simulink model "MBD_FOC_SENSORLESS_MODEL"  (R2022b)
settings: Solver=FixedStepDiscrete  StartTime=0.0  StopTime=9  FixedStep=.00005  RelTol=1e-3  EnableMultiTasking=on
PostLoadFcn:
  | MBD_FOC_SENSORLESS_DATA;
InitFcn:
  | MBD_FOC_SENSORLESS_DATA;
model workspace (MAT data in the model file):
  mwTaskManagerKernelLatency = 1e-06
values from neighbouring files (symbols this model uses):
  Iq_Ref_openLoop = 0.5    [MBD_FOC_SENSORLESS_DATA.m]
  PI_params = mcb.internal.SetControllerParameters(pmsm,inverter,PU_System,T_pwm,Ts,Ts_speed)    [MBD_FOC_SENSORLESS_DATA.m]
  PU_System = mcb_SetPUSystem(pmsm,inverter)    [MBD_FOC_SENSORLESS_DATA.m]
  PWM1max = 1600    [MBD_FOC_SENSORLESS_DATA.m]
  PWM_frequency = 20e3    (= 20000)    [MBD_FOC_SENSORLESS_DATA.m]
  Speed_Ref_openLoop = 500    [MBD_FOC_SENSORLESS_DATA.m]
  Ts = T_pwm    (= 5e-05)    [MBD_FOC_SENSORLESS_DATA.m]
  Ts_speed = 30*Ts    (= 0.0015)    [MBD_FOC_SENSORLESS_DATA.m]
undefined symbols (not defined in the file or in its folder): DiscIntNeverNeededParam, inverter, pmsm
libraries: mcbcontrolslib x9, simulink x4, slpidlib x3, mcbplantlib x1, autolibpmsmexterior x1
(part 2 of 2)

== system MBD_FOC_SENSORLESS_MODEL/Speed Control/Enable Switch/Codegen/Triggered Subsystem ==
  Trigger : TriggerPort  TriggerType=falling  VariantControl=Variant
  Data Store Write : DataStoreWrite  DataStoreName=Enable  IndexOptions=Index vector (dialog)  Indices=1  OutputSizes=1
  Delay : Delay  DelayLength=1  InitialCondition=0
  NOT : Logic  Operator=NOT  IconShape=distinctive  AllPortsSameDT=off  OutDataTypeStr=boolean
  wires:
  NOT/1 -> Data Store Write/1, Delay/1
  Delay/1 -> NOT/1

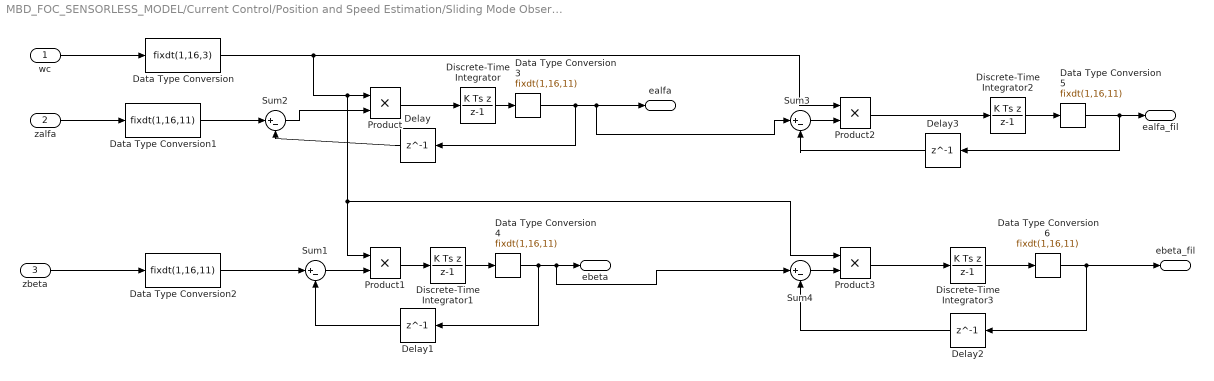
== system MBD_FOC_SENSORLESS_MODEL/Current Control/Position and Speed Estimation/Sliding Mode Observer/SMO Implemetation/Adaptive Filter1 ==
  wc : Inport
  zalfa : Inport  Port=2
  zbeta : Inport  Port=3
  Data Type Conversion : DataTypeConversion  OutDataTypeStr=fixdt(1,16,3)  SaturateOnIntegerOverflow=off  RndMeth=Floor
  Data Type Conversion{1..6} (6 alike) : DataTypeConversion  OutDataTypeStr=fixdt(1,16,11)  SaturateOnIntegerOverflow=off  RndMeth=Floor
  Delay{,1..3} (4 alike) : Delay  DelayLength=1
  Discrete-Time Integrator{,1..3} (4 alike) : DiscreteIntegrator  IntegratorMethod=Integration: Backward Euler  SampleTime=-1  OutDataTypeStr=fixdt(1,32,17)  ICPrevOutput=DiscIntNeverNeededParam  ICPrevScaledInput=DiscIntNeverNeededParam
  Product : Product  OutDataTypeStr=fixdt(1,32,14)
  Product1 : Product  OutDataTypeStr=fixdt(1,32,11)
  Product2 : Product
  Product3 : Product
  Sum{1..4} (4 alike) : Sum  Inputs=|+-
  ealfa : Outport  VectorParamsAs1DForOutWhenUnconnected=off
  ebeta : Outport  Port=2  VectorParamsAs1DForOutWhenUnconnected=off
  ealfa_fil : Outport  Port=3  VectorParamsAs1DForOutWhenUnconnected=off
  ebeta_fil : Outport  Port=4  VectorParamsAs1DForOutWhenUnconnected=off
  wires:
  Sum2/1 -> Product/2
  Product/1 -> Discrete-Time Integrator/1
  zalfa/1 -> Data Type Conversion1/1
  wc/1 -> Data Type Conversion/1
  Product1/1 -> Discrete-Time Integrator1/1
  Sum1/1 -> Product1/2
  zbeta/1 -> Data Type Conversion2/1
  Discrete-Time Integrator1/1 -> Data Type Conversion4/1
  Product2/1 -> Discrete-Time Integrator2/1
  Sum3/1 -> Product2/2
  Discrete-Time Integrator2/1 -> Data Type Conversion5/1
  Discrete-Time Integrator3/1 -> Data Type Conversion6/1
  Sum4/1 -> Product3/2
  Product3/1 -> Discrete-Time Integrator3/1
  Data Type Conversion/1 -> Product3/1, Product1/1, Product/1, Product2/1
  Data Type Conversion1/1 -> Sum2/1
  Data Type Conversion2/1 -> Sum1/1
  Discrete-Time Integrator/1 -> Data Type Conversion3/1
  Data Type Conversion3/1 -> Delay/1, Sum3/1, ealfa/1
  Data Type Conversion4/1 -> Delay1/1, Sum4/1, ebeta/1
  Delay/1 -> Sum2/2
  Delay1/1 -> Sum1/2
  Delay2/1 -> Sum4/2
  Delay3/1 -> Sum3/2
  Data Type Conversion5/1 -> ealfa_fil/1, Delay3/1
  Data Type Conversion6/1 -> ebeta_fil/1, Delay2/1

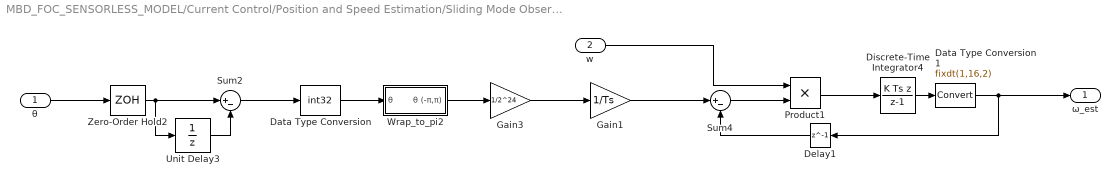
== system MBD_FOC_SENSORLESS_MODEL/Current Control/Position and Speed Estimation/Sliding Mode Observer/SMO Implemetation/Subsystem ==
  θ : Inport
  w : Inport  Port=2
  Data Type Conversion : DataTypeConversion  OutDataTypeStr=int32  ConvertRealWorld=Stored Integer (SI)  SaturateOnIntegerOverflow=off  RndMeth=Floor
  Data Type Conversion1 : DataTypeConversion  OutDataTypeStr=fixdt(1,16,2)  SaturateOnIntegerOverflow=off  RndMeth=Floor
  Delay1 : Delay  DelayLength=1
  Discrete-Time Integrator4 : DiscreteIntegrator  IntegratorMethod=Integration: Backward Euler  SampleTime=-1  OutDataTypeStr=fixdt(1,32,8)  ICPrevOutput=DiscIntNeverNeededParam  ICPrevScaledInput=DiscIntNeverNeededParam
  Gain1 : Gain  Gain=1/Ts  OutDataTypeStr=fixdt(1,16,3)
  Gain3 : Gain  Gain=1/2^24  OutDataTypeStr=fixdt(1,16,12)
  Product1 : Product  OutDataTypeStr=fixdt(1,32,8)
  Sum2 : Sum  Inputs=|+-  AccumDataTypeStr=fixdt(1,16,12)  OutDataTypeStr=fixdt(1,32,24)
  Sum4 : Sum  Inputs=|+-
  Unit Delay3 : UnitDelay  SampleTime=Ts  HasFrameUpgradeWarning=on
  Wrap_to_pi2 : Subsystem  VariantControl=VSS_STD
  Zero-Order Hold2 : ZeroOrderHold  SampleTime=Ts
  ω_est : Outport  VectorParamsAs1DForOutWhenUnconnected=off
  wires:
  Unit Delay3/1 -> Sum2/2
  Zero-Order Hold2/1 -> Sum2/1, Unit Delay3/1
  Wrap_to_pi2/1(θ (-π,π)) -> Gain3/1
  Sum4/1 -> Product1/2
  Product1/1 -> Discrete-Time Integrator4/1
  θ/1 -> Zero-Order Hold2/1
  Gain1/1 -> Sum4/1
  Delay1/1 -> Sum4/2
  Sum2/1 -> Data Type Conversion/1
  Data Type Conversion/1 -> Wrap_to_pi2/1(θ)
  Gain3/1 -> Gain1/1
  Discrete-Time Integrator4/1 -> Data Type Conversion1/1
  w/1 -> Product1/1
  Data Type Conversion1/1 -> Delay1/1, ω_est/1

== system MBD_FOC_SENSORLESS_MODEL/Current Control/Position and Speed Estimation/Sliding Mode Observer/SMO Implemetation/atan2 ==
  note: Consistent with Microchip notation:
      |
      | x_α = cos(θ) * x_d - sin(θ) * x_q
      | x_β = sin(θ) * x_d + cos(θ) * x_q
      |
      | θ = atan2(sin(θ)/cos(θ)) = atan2(-x_α/x_β)
      |
      | provided x_d = 0, which is true in case of E_d
  α : Inport
  β : Inport  Port=2
  Bias2 : Bias  Bias=(pi/4)+(pi/4)  SaturateOnIntegerOverflow=off
  Data Type Conversion3 : DataTypeConversion  OutDataTypeStr=fixdt(1,16,12)  SaturateOnIntegerOverflow=off  RndMeth=Floor
  Data Type Conversion4 : DataTypeConversion  OutDataTypeStr=uint16  ConvertRealWorld=Stored Integer (SI)  SaturateOnIntegerOverflow=off  RndMeth=Floor
  Gain2 : Gain  Gain=1/2^12  OutDataTypeStr=fixdt(1,16,12)
  Gain3 : Gain  Gain=-1  OutDataTypeStr=Inherit: Same as input
  Subsystem1 : Subsystem
  Trigonometric Function : Trigonometry  Operator=atan2  ApproximationMethod=CORDIC
  Wrap_to_pi1 : Subsystem  VariantControl=VSS_STD
  θ : Outport  VectorParamsAs1DForOutWhenUnconnected=off
  wires:
  Trigonometric Function/1 -> Data Type Conversion3/1
  Gain3/1 -> Trigonometric Function/1
  α/1 -> Gain3/1
  β/1 -> Trigonometric Function/2
  Data Type Conversion3/1 -> Subsystem1/1(theta(-pi,pi))
  Subsystem1/1(theta(0,2pi)) -> Bias2/1
  Bias2/1 -> Data Type Conversion4/1
  Data Type Conversion4/1 -> Wrap_to_pi1/1(θ)
  Wrap_to_pi1/1(θ (0,2π)) -> Gain2/1  "z"
  Gain2/1 -> θ/1

== system MBD_FOC_SENSORLESS_MODEL/Current Control/Position and Speed Estimation/Sliding Mode Observer/SMO Implemetation/Subsystem/Wrap_to_pi2 ==
  note: What's left after
      | division by 2pi
  note: This block limits the output angle between +/- π.
  note: Add pi
  note: What's left after
      | division by 2pi
      | again
  note: Subtract pi
  θ : Inport
  Bias : Bias  Bias=pi*16777216  SaturateOnIntegerOverflow=off
  Bias1 : Bias  Bias=-pi*16777216  SaturateOnIntegerOverflow=off
  Math Function : Math  Operator=mod  SignedPower=on
  Math Function1 : Math  Operator=mod  SignedPower=on
  load torque1 : Constant  Value=2*pi*16777216  OutDataTypeStr=int32  SampleTime=Ts
  θ (-π,π) : Outport  VectorParamsAs1DForOutWhenUnconnected=off
  wires:
  Math Function1/1 -> Bias/1
  θ/1 -> Math Function1/1
  Math Function/1 -> Bias1/1
  load torque1/1 -> Math Function1/2, Math Function/2
  Bias/1 -> Math Function/1
  Bias1/1 -> θ (-π,π)/1

== system MBD_FOC_SENSORLESS_MODEL/Current Control/Position and Speed Estimation/Sliding Mode Observer/SMO Implemetation/atan2/Subsystem1 ==
  theta(-pi,pi) : Inport
  2pi : Constant  Value=2*pi  OutDataTypeStr=fixdt(1,16,12)  SampleTime=Ts  mask(TL_Constant){data={'date',734873.5078369329}}
      settings: CopyFcn=if exist('tl_reset_reviewflag','file')==2,tl_reset_reviewflag(gcbh);end  DeleteFcn=if exist('delete_tlblock','file')==2,delete_tlblock(gcbh);end  NameChangeFcn=if exist('rename_tlblock','file')==2,rename_tlblock(gcbh);end  OpenFcn=if exist('tl_open_blockdlg','file')==2,tl_open_blockdlg(gcbh);else,open_system(gcbh,'parameter');end
      mask Help: eval(['if exist(''tl_online_help'',''file'') == 2, tl_online_help(''Topic'',''TL_Constant''),else, web([''jar:file:///'',matlabroot,''/help/toolbox/simulink/help.jar!/slref/' lower(get_param(gcbh,'Blocktype')) '.html''], ''-helpbrowser''),end'])
      mask Display: plot([-0.05, 1.05, NaN, -0.05, 1.05],[.01, .01, NaN, .99, .99])
  Sum : Sum
  Switch2 : Switch  Criteria=u2 > Threshold  SaturateOnIntegerOverflow=off  InputSameDT=off
  theta(0,2pi) : Outport  VectorParamsAs1DForOutWhenUnconnected=off
  wires:
  2pi/1 -> Sum/2
  theta(-pi,pi)/1 -> Sum/1, Switch2/2, Switch2/1
  Sum/1 -> Switch2/3  "err"
  Switch2/1 -> theta(0,2pi)/1

== system MBD_FOC_SENSORLESS_MODEL/Current Control/Position and Speed Estimation/Sliding Mode Observer/SMO Implemetation/atan2/Wrap_to_pi1 ==
  note: This block limits the output angle between 0 to 2π.
  θ : Inport
  Math Function : Math  Operator=rem  SignedPower=on
  load torque2 : Constant  Value=2*pi*2^12  OutDataTypeStr=uint16  SampleTime=Ts
  θ (0,2π) : Outport  VectorParamsAs1DForOutWhenUnconnected=off
  wires:
  Math Function/1 -> θ (0,2π)/1
  θ/1 -> Math Function/1
  load torque2/1 -> Math Function/2

== stateflow chart MBD_FOC_SENSORLESS_MODEL/Current Control/Position and Speed Estimation/OpentoClosed/Chart ==
  state Init
    during: Mode = 0;
    SpeedCtrl = 0;
  state Align
    during: Mode = 0;
    SpeedCtrl = 0;
  state ClosedLoopFilter
    during: Mode = 2;
    SpeedCtrl = 1;
  state ClosedLoop
    during: Mode = 2;
    SpeedCtrl = 0;
  state OpenLoop
    during: Mode = 1;
    SpeedCtrl = 0;
  (default) -> Init
  ClosedLoopFilter -> Init : [En == 0]
  ClosedLoop -> Init [order 1] : [En == 0]
  Init -> Align : [En == 1]
  Align -> Init [order 1] : [En == 0]
  OpenLoop -> Init [order 2] : [En == 0]
  Align -> OpenLoop [order 2] : after(0.5,sec)
  ClosedLoop -> ClosedLoopFilter [order 2] : after(0.1,sec)
  OpenLoop -> ClosedLoop [order 1] : after(2,sec)[SpeedFb > Limit]
  data: Limit input fixdt(1,16,14); SpeedFb input fixdt(1,16,14); Mode output uint16; En input boolean; SpeedCtrl output uint16
